simulink model "Task5_Sine_Wave_Control_Flow"  (R2024b)
settings: Solver=VariableStepAuto  StartTime=0.0  StopTime=10.0  RelTol=1e-3
settings Model: Creator=Ahmad  LastModifiedBy=Ahmad

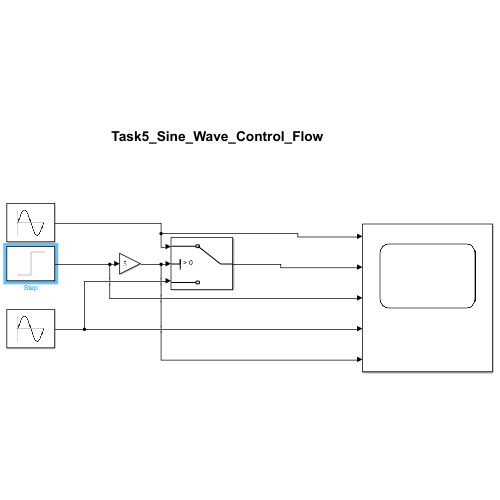
[thumbnail: Simulink's stored preview of the top-level diagram]
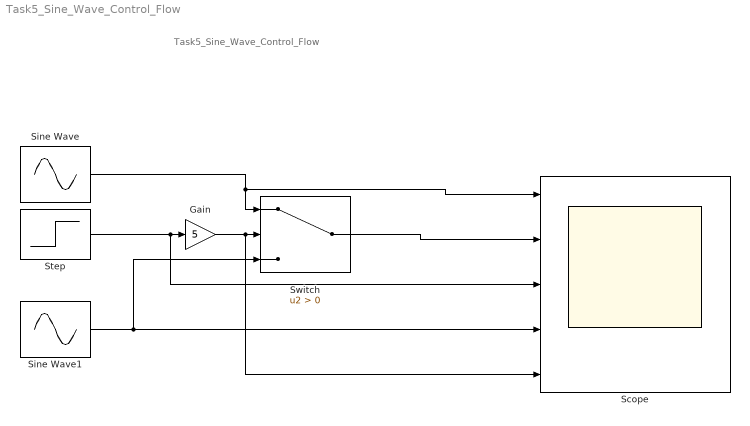
== system Task5_Sine_Wave_Control_Flow ==
  note: Task5_Sine_Wave_Control_Flow
  Gain : Gain  Gain=5
  Scope : Scope  NumInputPorts=5
  Sine Wave : Sin  SampleTime=0
  Sine Wave1 : Sin  Phase=-pi  SampleTime=0
  Step : Step  Time=2  SampleTime=0
  Switch : Switch  Criteria=u2 > Threshold  SaturateOnIntegerOverflow=off  InputSameDT=off
  wires:
  Step/1 -> Scope/3, Gain/1
  Sine Wave/1 -> Switch/1, Scope/1
  Sine Wave1/1 -> Switch/3, Scope/4
  Switch/1 -> Scope/2
  Gain/1 -> Scope/5, Switch/2
